simulink library "jcc"  (Simulink 8.1)
settings: Solver=ode1  StartTime=0.0  StopTime=Inf  FixedStep=0.001  RelTol=1e-3
PostLoadFcn:
  | , if any(exist('dsrtsu_mdlpostloadfcn', 'file') == [2, 3, 6]), try dsrtsu_mdlpostloadfcn('Execute', bdroot); catch fprintf('Error in PostLoadFcn (dsrtsu_mdlpostloadfcn) for model "%s":\n %s\n', bdroot, lasterr); end, end,
libraries: cav x1, cda x1, cec x1, cor x1, crf x1, ccs x1, cct x1, csr x1, css x1, crs x1
settings Model: DSRTSU_INTERNAL_RTI_VER=450  DSRTSU_INTERNAL_RTI_TYPE=rti1401  RTICANMMDATA=struct('GeneralSetupData',struct('modelroot','D:\ELN150201_TAIWAN\trunk\AdasDragon\software\sw_development\arch\app\jud','generalsettings',struct('filesettings',struct('destfolder',struct('Name','RTICANMM_FILES','Check',1),'buildfolder',struct('Name','.','Check',1),'AbsDestfolder',struct('Name','D:\ELN150201_TAIWAN\trunk\AdasDragon\software\sw_development\arch\app\jud\RTICANMM_FILES'),'AbsBuildfolder',struct('Name','D:\ELN150201_TAIWAN\trunk\AdasDragon\software\sw_development\arch\app\jud'))),'options',struct('addpaths',1,'rmpaths',1,'addtrcexclusion',logical(1),'cannavigator',struct('checkmonitoring',0),'show_usrtrc',0,'use_usrtrc',0),'advanced',struct('options',[1 1 1 1 1 1 1 1 1 1 1 1 1 1 1 1 1 1 1 1 1 1 1 1 1 1 1 1 1 1 1 1 1 1 1 1 1 1 1 1 1 1 1 1 1 1 1 1 1 1 1 1 1 1 1 1 1 1 1 1 1 1 1 1 1 1 1 1 1 1 1 1 1 1 1 1 1 1 1 1 1 1 1 1 1 1 1 1 1 1 1 1 1 1 1 1 1 1 1 1]),'MPSetup',{{}},'modelname','jcc','block','jcc'))  DSRTSU_INTERNAL_RTIFPGA=40  Creator=AT015411  LastModifiedBy=AT015555

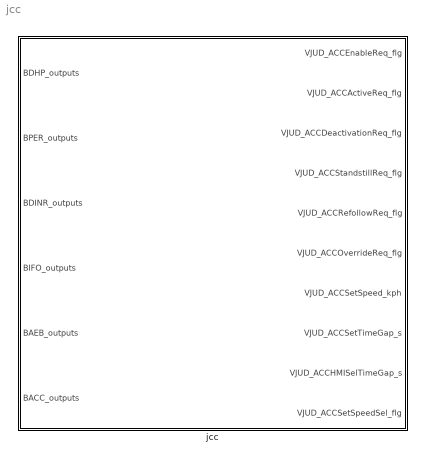
== system jcc ==
  jcc : Subsystem

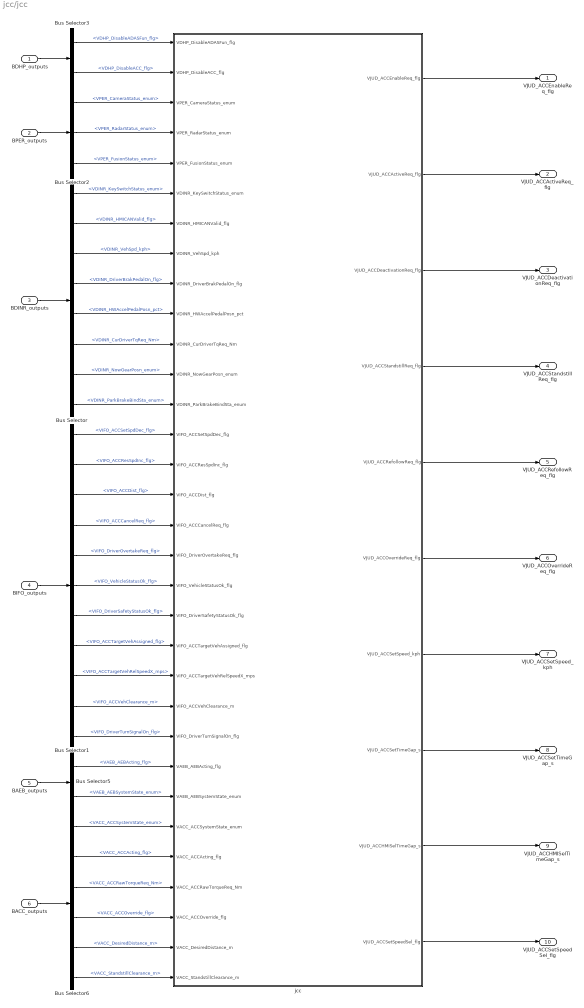
== system jcc/jcc ==
  BDHP_outputs : Inport  OutDataTypeStr=Bus: BDHP_outputs
  BPER_outputs : Inport  Port=2  OutDataTypeStr=Bus: BPER_outputs
  BDINR_outputs : Inport  Port=3  OutDataTypeStr=Bus: BDINR_outputs
  BIFO_outputs : Inport  Port=4  OutDataTypeStr=Bus: BIFO_outputs
  BAEB_outputs : Inport  Port=5  OutDataTypeStr=Bus: BAEB_outputs
  BACC_outputs : Inport  Port=6  OutDataTypeStr=Bus: BACC_outputs
  Bus Selector : BusSelector  OutputSignals=VDINR_KeySwitchStatus_enum,VDINR_HMICANValid_flg,VDINR_VehSpd_kph,VDINR_DriverBrakPedalOn_flg,VDINR_HWAccelPedalPosn_pct,VDINR_CurDriverTqReq_Nm,VDINR_NowGearPosn_enum,VDINR_ParkBrakeBindSta_enum
  Bus Selector1 : BusSelector  OutputSignals=VIFO_ACCSetSpdDec_flg,VIFO_ACCResSpdInc_flg,VIFO_ACCDist_flg,VIFO_ACCCancelReq_flg,VIFO_DriverOvertakeReq_flg,VIFO_VehicleStatusOk_flg,VIFO_DriverSafetyStatusOk_flg,VIFO_ACCTargetVehAssigned_flg,VIFO_ACCTargetVehRelSpeedX_mps,VIFO_ACCVehClearance_m,VIFO_DriverTurnSignalOn_flg
  Bus Selector2 : BusSelector  OutputSignals=VPER_CameraStatus_enum,VPER_RadarStatus_enum,VPER_FusionStatus_enum
  Bus Selector3 : BusSelector  OutputSignals=VDHP_DisableADASFun_flg,VDHP_DisableACC_flg
  Bus Selector5 : BusSelector  OutputSignals=VAEB_AEBActing_flg,VAEB_AEBSystemState_enum
  Bus Selector6 : BusSelector  OutputSignals=VACC_ACCSystemState_enum,VACC_ACCActing_flg,VACC_ACCRawTorqueReq_Nm,VACC_ACCOverride_flg,VACC_DesiredDistance_m,VACC_StandstillClearance_m
  jcc : Subsystem
  VJUD_ACCEnableReq_flg : Outport
  VJUD_ACCActiveReq_flg : Outport  Port=2
  VJUD_ACCDeactivationReq_flg : Outport  Port=3
  VJUD_ACCStandstillReq_flg : Outport  Port=4
  VJUD_ACCRefollowReq_flg : Outport  Port=5
  VJUD_ACCOverrideReq_flg : Outport  Port=6
  VJUD_ACCSetSpeed_kph : Outport  Port=7
  VJUD_ACCSetTimeGap_s : Outport  Port=8
  VJUD_ACCHMISelTimeGap_s : Outport  Port=9
  VJUD_ACCSetSpeedSel_flg : Outport  Port=10
  wires:
  Bus Selector1/11 -> jcc/24(VIFO_DriverTurnSignalOn_flg)  "<VIFO_DriverTurnSignalOn_flg>"
  Bus Selector6/6 -> jcc/32(VACC_StandstillClearance_m)  "<VACC_StandstillClearance_m>"
  Bus Selector6/5 -> jcc/31(VACC_DesiredDistance_m)  "<VACC_DesiredDistance_m>"
  Bus Selector6/4 -> jcc/30(VACC_ACCOverride_flg)  "<VACC_ACCOverride_flg>"
  Bus Selector6/3 -> jcc/29(VACC_ACCRawTorqueReq_Nm)  "<VACC_ACCRawTorqueReq_Nm>"
  BIFO_outputs/1 -> Bus Selector1/1
  BPER_outputs/1 -> Bus Selector2/1
  BDHP_outputs/1 -> Bus Selector3/1
  BACC_outputs/1 -> Bus Selector6/1
  jcc/1(VJUD_ACCEnableReq_flg) -> VJUD_ACCEnableReq_flg/1
  Bus Selector5/1 -> jcc/25(VAEB_AEBActing_flg)  "<VAEB_AEBActing_flg>"
  Bus Selector3/1 -> jcc/1(VDHP_DisableADASFun_flg)  "<VDHP_DisableADASFun_flg>"
  Bus Selector3/2 -> jcc/2(VDHP_DisableACC_flg)  "<VDHP_DisableACC_flg>"
  Bus Selector2/1 -> jcc/3(VPER_CameraStatus_enum)  "<VPER_CameraStatus_enum>"
  Bus Selector2/2 -> jcc/4(VPER_RadarStatus_enum)  "<VPER_RadarStatus_enum>"
  Bus Selector2/3 -> jcc/5(VPER_FusionStatus_enum)  "<VPER_FusionStatus_enum>"
  jcc/6(VJUD_ACCOverrideReq_flg) -> VJUD_ACCOverrideReq_flg/1
  jcc/5(VJUD_ACCRefollowReq_flg) -> VJUD_ACCRefollowReq_flg/1
  jcc/4(VJUD_ACCStandstillReq_flg) -> VJUD_ACCStandstillReq_flg/1
  jcc/3(VJUD_ACCDeactivationReq_flg) -> VJUD_ACCDeactivationReq_flg/1
  jcc/2(VJUD_ACCActiveReq_flg) -> VJUD_ACCActiveReq_flg/1
  jcc/7(VJUD_ACCSetSpeed_kph) -> VJUD_ACCSetSpeed_kph/1
  jcc/8(VJUD_ACCSetTimeGap_s) -> VJUD_ACCSetTimeGap_s/1
  jcc/10(VJUD_ACCSetSpeedSel_flg) -> VJUD_ACCSetSpeedSel_flg/1
  Bus Selector6/1 -> jcc/27(VACC_ACCSystemState_enum)  "<VACC_ACCSystemState_enum>"
  BAEB_outputs/1 -> Bus Selector5/1
  Bus Selector6/2 -> jcc/28(VACC_ACCActing_flg)  "<VACC_ACCActing_flg>"
  Bus Selector1/6 -> jcc/19(VIFO_VehicleStatusOk_flg)  "<VIFO_VehicleStatusOk_flg>"
  Bus Selector1/5 -> jcc/18(VIFO_DriverOvertakeReq_flg)  "<VIFO_DriverOvertakeReq_flg>"
  Bus Selector1/7 -> jcc/20(VIFO_DriverSafetyStatusOk_flg)  "<VIFO_DriverSafetyStatusOk_flg>"
  Bus Selector1/4 -> jcc/17(VIFO_ACCCancelReq_flg)  "<VIFO_ACCCancelReq_flg>"
  BDINR_outputs/1 -> Bus Selector/1
  Bus Selector/1 -> jcc/6(VDINR_KeySwitchStatus_enum)  "<VDINR_KeySwitchStatus_enum>"
  Bus Selector/7 -> jcc/12(VDINR_NowGearPosn_enum)  "<VDINR_NowGearPosn_enum>"
  Bus Selector/2 -> jcc/7(VDINR_HMICANValid_flg)  "<VDINR_HMICANValid_flg>"
  Bus Selector/3 -> jcc/8(VDINR_VehSpd_kph)  "<VDINR_VehSpd_kph>"
  Bus Selector/4 -> jcc/9(VDINR_DriverBrakPedalOn_flg)  "<VDINR_DriverBrakPedalOn_flg>"
  Bus Selector/5 -> jcc/10(VDINR_HWAccelPedalPosn_pct)  "<VDINR_HWAccelPedalPosn_pct>"
  Bus Selector/6 -> jcc/11(VDINR_CurDriverTqReq_Nm)  "<VDINR_CurDriverTqReq_Nm>"
  Bus Selector/8 -> jcc/13(VDINR_ParkBrakeBindSta_enum)  "<VDINR_ParkBrakeBindSta_enum>"
  Bus Selector1/1 -> jcc/14(VIFO_ACCSetSpdDec_flg)  "<VIFO_ACCSetSpdDec_flg>"
  Bus Selector1/2 -> jcc/15(VIFO_ACCResSpdInc_flg)  "<VIFO_ACCResSpdInc_flg>"
  Bus Selector1/3 -> jcc/16(VIFO_ACCDist_flg)  "<VIFO_ACCDist_flg>"
  jcc/9(VJUD_ACCHMISelTimeGap_s) -> VJUD_ACCHMISelTimeGap_s/1
  Bus Selector5/2 -> jcc/26(VAEB_AEBSystemState_enum)  "<VAEB_AEBSystemState_enum>"
  Bus Selector1/8 -> jcc/21(VIFO_ACCTargetVehAssigned_flg)  "<VIFO_ACCTargetVehAssigned_flg>"
  Bus Selector1/9 -> jcc/22(VIFO_ACCTargetVehRelSpeedX_mps)  "<VIFO_ACCTargetVehRelSpeedX_mps>"
  Bus Selector1/10 -> jcc/23(VIFO_ACCVehClearance_m)  "<VIFO_ACCVehClearance_m>"

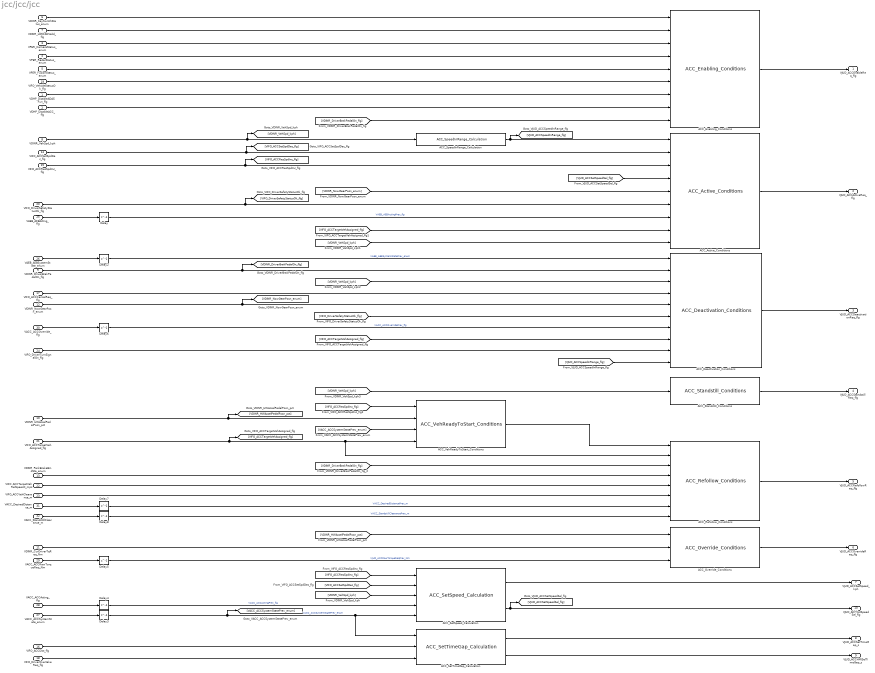
== system jcc/jcc/jcc ==
  VDHP_DisableADASFun_flg : Inport
  VDHP_DisableACC_flg : Inport  Port=2
  VPER_CameraStatus_enum : Inport  Port=3
  VPER_RadarStatus_enum : Inport  Port=4
  VPER_FusionStatus_enum : Inport  Port=5
  VDINR_KeySwitchStatus_enum : Inport  Port=6
  VDINR_HMICANValid_flg : Inport  Port=7
  VDINR_VehSpd_kph : Inport  Port=8
  VDINR_DriverBrakPedalOn_flg : Inport  Port=9
  VDINR_HWAccelPedalPosn_pct : Inport  Port=10
  VDINR_CurDriverTqReq_Nm : Inport  Port=11
  VDINR_NowGearPosn_enum : Inport  Port=12
  VDINR_ParkBrakeBindSta_enum : Inport  Port=13
  VIFO_ACCSetSpdDec_flg : Inport  Port=14
  VIFO_ACCResSpdInc_flg : Inport  Port=15
  VIFO_ACCDist_flg : Inport  Port=16
  VIFO_ACCCancelReq_flg : Inport  Port=17
  VIFO_DriverOvertakeReq_flg : Inport  Port=18
  VIFO_VehicleStatusOk_flg : Inport  Port=19
  VIFO_DriverSafetyStatusOk_flg : Inport  Port=20
  VIFO_ACCTargetVehAssigned_flg : Inport  Port=21
  VIFO_ACCTargetVehRelSpeedX_mps : Inport  Port=22
  VIFO_ACCVehClearance_m : Inport  Port=23
  VIFO_DriverTurnSignalOn_flg : Inport  Port=24
  VAEB_AEBActing_flg : Inport  Port=25
  VAEB_AEBSystemState_enum : Inport  Port=26
  VACC_ACCSystemState_enum : Inport  Port=27
  VACC_ACCActing_flg : Inport  Port=28
  VACC_ACCRawTorqueReq_Nm : Inport  Port=29
  VACC_ACCOverride_flg : Inport  Port=30
  VACC_DesiredDistance_m : Inport  Port=31
  VACC_StandstillClearance_m : Inport  Port=32
  ACC_Active_Conditions : cav/ACC_Active_Conditions
  ACC_Deactivation_Conditions : cda/ACC_Deactivation_Conditions
  ACC_Enabling_Conditions : cec/ACC_Enabling_Conditions
  ACC_Override_Conditions : cor/ACC_Override_Conditions
  ACC_Refollow_Conditions : crf/ACC_Refollow_Conditions
  ACC_SetSpeed_Calculation : ccs/ACC_SetSpeed_Calculation
  ACC_SetTimeGap_Calculation : cct/ACC_SetTimeGap_Calculation
  ACC_SpeedInRange_Calculation : csr/ACC_SpeedInRange_Calculation
  ACC_Standstill_Conditions : css/ACC_Standstill_Conditions
  ACC_VehReadyToStart_Conditions : crs/ACC_VehReadyToStart_Conditions
  Delay{,2..8} (8 alike) : Delay  DelayLength=1  InitialCondition=0
  VJUD_ACCEnableReq_flg : Outport
  VJUD_ACCActiveReq_flg : Outport  Port=2
  VJUD_ACCDeactivationReq_flg : Outport  Port=3
  VJUD_ACCStandstillReq_flg : Outport  Port=4
  VJUD_ACCRefollowReq_flg : Outport  Port=5
  VJUD_ACCOverrideReq_flg : Outport  Port=6
  VJUD_ACCSetSpeed_kph : Outport  Port=7
  VJUD_ACCSetTimeGap_s : Outport  Port=8
  VJUD_ACCHMISelTimeGap_s : Outport  Port=9
  VJUD_ACCSetSpeedSel_flg : Outport  Port=10
  wires:
  Delay5/1 -> ACC_Override_Conditions/3  "VJUD_ACCRawTorqueReqPrev_Nm"
  VACC_ACCRawTorqueReq_Nm/1 -> Delay5/1
  VDINR_VehSpd_kph/1 -> [VDINR_VehSpd_kph], ACC_SpeedInRange_Calculation/1
  ACC_SpeedInRange_Calculation/1 -> [VJUD_ACCSpeedInRange_flg], ACC_Active_Conditions/1
  ACC_Enabling_Conditions/1 -> VJUD_ACCEnableReq_flg/1
  ACC_Active_Conditions/1 -> VJUD_ACCActiveReq_flg/1
  ACC_Deactivation_Conditions/1 -> VJUD_ACCDeactivationReq_flg/1
  ACC_Standstill_Conditions/1 -> VJUD_ACCStandstillReq_flg/1
  ACC_Refollow_Conditions/1 -> VJUD_ACCRefollowReq_flg/1
  ACC_VehReadyToStart_Conditions/1 -> ACC_Refollow_Conditions/1
  ACC_Override_Conditions/1 -> VJUD_ACCOverrideReq_flg/1
  [VJUD_ACCSetSpeedSel_flg] -> ACC_Active_Conditions/4
  VDINR_KeySwitchStatus_enum/1 -> ACC_Enabling_Conditions/1
  VIFO_VehicleStatusOk_flg/1 -> ACC_Enabling_Conditions/6
  VDINR_HMICANValid_flg/1 -> ACC_Enabling_Conditions/2
  VPER_CameraStatus_enum/1 -> ACC_Enabling_Conditions/3
  VPER_RadarStatus_enum/1 -> ACC_Enabling_Conditions/4
  VPER_FusionStatus_enum/1 -> ACC_Enabling_Conditions/5
  VDHP_DisableADASFun_flg/1 -> ACC_Enabling_Conditions/7
  VDHP_DisableACC_flg/1 -> ACC_Enabling_Conditions/8
  [VDINR_VehSpd_kph] -> ACC_Standstill_Conditions/1
  Delay/1 -> ACC_Active_Conditions/7  "VAEB_AEBActingPrev_flg"
  VDINR_DriverBrakPedalOn_flg/1 -> [VDINR_DriverBrakPedalOn_flg], ACC_Deactivation_Conditions/2
  [VDINR_DriverBrakPedalOn_flg] -> ACC_Refollow_Conditions/3
  VDINR_CurDriverTqReq_Nm/1 -> ACC_Override_Conditions/2
  VDINR_HWAccelPedalPosn_pct/1 -> [VDINR_HWAccelPedalPosn_pct], ACC_VehReadyToStart_Conditions/2
  ACC_SetSpeed_Calculation/1 -> VJUD_ACCSetSpeed_kph/1
  ACC_SetTimeGap_Calculation/1 -> VJUD_ACCSetTimeGap_s/1
  VAEB_AEBActing_flg/1 -> Delay/1
  Delay3/1 -> ACC_SetTimeGap_Calculation/1, ACC_SetSpeed_Calculation/5, [VACC_ACCSystemStatePrev_enum]  "VACC_ACCSystemStatePrev_enum"
  ACC_SetSpeed_Calculation/2 -> [VJUD_ACCSetSpeedSel_flg], VJUD_ACCSetSpeedSel_flg/1
  [VIFO_ACCResSpdInc_flg] -> ACC_VehReadyToStart_Conditions/1
  VACC_ACCSystemState_enum/1 -> Delay3/1
  [VDINR_DriverBrakPedalOn_flg] -> ACC_Enabling_Conditions/9
  VACC_ACCActing_flg/1 -> Delay4/1
  [VDINR_VehSpd_kph] -> ACC_SetSpeed_Calculation/3
  Delay4/1 -> ACC_SetSpeed_Calculation/4  "VACC_ACCActingPrev_flg"
  VIFO_ACCSetSpdDec_flg/1 -> ACC_Active_Conditions/2, [VIFO_ACCSetSpdDec_flg]
  VIFO_ACCResSpdInc_flg/1 -> ACC_Active_Conditions/3, [VIFO_ACCResSpdInc_flg]
  [VIFO_ACCResSpdInc_flg] -> ACC_SetSpeed_Calculation/1
  [VIFO_ACCSetSpdDec_flg] -> ACC_SetSpeed_Calculation/2
  VIFO_DriverOvertakeReq_flg/1 -> ACC_SetTimeGap_Calculation/3
  VIFO_ACCDist_flg/1 -> ACC_SetTimeGap_Calculation/2
  [VDINR_VehSpd_kph] -> ACC_Deactivation_Conditions/3
  VIFO_ACCCancelReq_flg/1 -> ACC_Deactivation_Conditions/4
  VDINR_NowGearPosn_enum/1 -> ACC_Deactivation_Conditions/5, [VDINR_NowGearPosn_enum]
  VIFO_DriverSafetyStatusOk_flg/1 -> ACC_Active_Conditions/6, [VIFO_DriverSafetyStatusOk_flg]
  [VDINR_NowGearPosn_enum] -> ACC_Active_Conditions/5
  [VIFO_DriverSafetyStatusOk_flg] -> ACC_Deactivation_Conditions/6
  VDINR_ParkBrakeBindSta_enum/1 -> ACC_Refollow_Conditions/4
  [VDINR_HWAccelPedalPosn_pct] -> ACC_Override_Conditions/1
  ACC_SetTimeGap_Calculation/2 -> VJUD_ACCHMISelTimeGap_s/1
  VAEB_AEBSystemState_enum/1 -> Delay2/1
  Delay2/1 -> ACC_Deactivation_Conditions/1  "VAEB_AEBSystemStatePrev_enum"
  VACC_ACCOverride_flg/1 -> Delay6/1
  Delay6/1 -> ACC_Deactivation_Conditions/7  "VACC_ACCOverridePrev_flg"
  [VACC_ACCSystemStatePrev_enum] -> ACC_VehReadyToStart_Conditions/3
  VIFO_ACCTargetVehAssigned_flg/1 -> [VIFO_ACCTargetVehAssigned_flg], ACC_VehReadyToStart_Conditions/4, ACC_Refollow_Conditions/2
  VIFO_ACCTargetVehRelSpeedX_mps/1 -> ACC_Refollow_Conditions/5
  VIFO_ACCVehClearance_m/1 -> ACC_Refollow_Conditions/6
  VACC_DesiredDistance_m/1 -> Delay7/1
  Delay7/1 -> ACC_Refollow_Conditions/7  "VACC_DesiredDistancePrev_m"
  [VIFO_ACCTargetVehAssigned_flg] -> ACC_Deactivation_Conditions/8
  [VIFO_ACCTargetVehAssigned_flg] -> ACC_Active_Conditions/8
  [VDINR_VehSpd_kph] -> ACC_Active_Conditions/9
  VACC_StandstillClearance_m/1 -> Delay8/1
  Delay8/1 -> ACC_Refollow_Conditions/8  "VACC_StandstillClearancePrev_m"
  VIFO_DriverTurnSignalOn_flg/1 -> ACC_Deactivation_Conditions/9
  [VJUD_ACCSpeedInRange_flg] -> ACC_Deactivation_Conditions/10
